simulink model "PI_Controller"  (R2020b)
settings: Solver=VariableStepAuto  StartTime=0.0  StopTime=10  RelTol=1e-3
values from neighbouring files (symbols this model uses):
  Ki = 40    [Variables.m]
  Kp = 800    [Variables.m]
settings Model: DataDictionary=cruise_control_data.sldd  Creator=dell  LastModifiedBy=dell
settings DataIOCC: SaveOutput=off  SaveTime=off

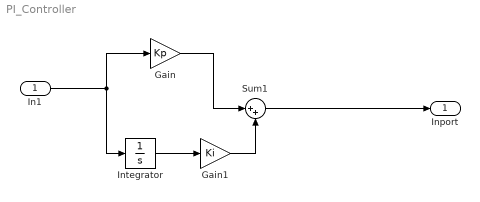
== system PI_Controller ==
  In1 : Inport  OutDataTypeStr=double  PortDimensions=1  SampleTime=0
  Gain : Gain  Gain=Kp
  Gain1 : Gain  Gain=Ki
  Integrator : Integrator
  Sum1 : Sum  Inputs=|++
  Inport : Outport  OutDataTypeStr=double  PortDimensions=1  SampleTime=0
  wires:
  In1/1 -> Gain/1, Integrator/1
  Integrator/1 -> Gain1/1
  Sum1/1 -> Inport/1
  Gain1/1 -> Sum1/2
  Gain/1 -> Sum1/1
